simulink model "LQR_Controller"  (R2020b)
settings: Solver=VariableStepAuto  StartTime=0.0  StopTime=10.0  RelTol=1e-3
settings Model: Creator=24365  LastModifiedBy=24365

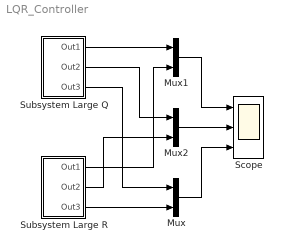
== system LQR_Controller ==
  Mux : Mux  Inputs=2
  Mux1 : Mux  Inputs=2
  Mux2 : Mux  Inputs=2
  Scope : Scope  NumInputPorts=3
  Subsystem Large Q : Subsystem
  Subsystem Large R : Subsystem
  wires:
  Subsystem Large Q/1(Out1) -> Mux1/1
  Subsystem Large Q/2(Out2) -> Mux2/1
  Subsystem Large Q/3(Out3) -> Mux/1
  Subsystem Large R/1(Out1) -> Mux1/2
  Subsystem Large R/2(Out2) -> Mux2/2
  Subsystem Large R/3(Out3) -> Mux/2
  Mux1/1 -> Scope/1
  Mux2/1 -> Scope/2
  Mux/1 -> Scope/3

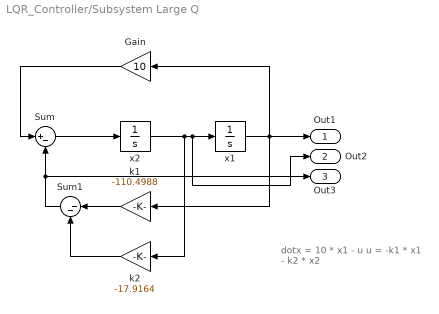
== system LQR_Controller/Subsystem Large Q ==
  note: dotx = 10 * x1 - u
      | u = -k1 * x1 - k2 * x2
  Gain : Gain  Gain=10
  Sum : Sum  Inputs=|+-
  Sum1 : Sum  Inputs=|--
  k1 : Gain  Gain=-110.4988
  k2 : Gain  Gain=-17.9164
  x1 : Integrator  InitialCondition=5
  x2 : Integrator
  Out1 : Outport
  Out2 : Outport  Port=2
  Out3 : Outport  Port=3
  wires:
  x2/1 -> k2/1, Out2/1, x1/1
  Sum1/1 -> Out3/1, Sum/2
  k2/1 -> Sum1/2
  k1/1 -> Sum1/1
  Gain/1 -> Sum/1
  x1/1 -> Out1/1, k1/1, Gain/1
  Sum/1 -> x2/1

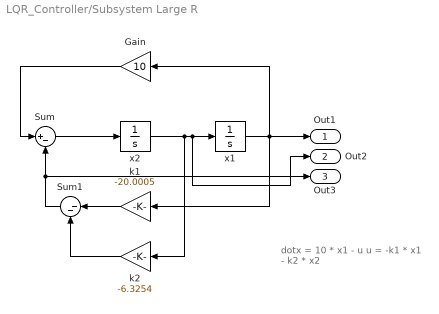
== system LQR_Controller/Subsystem Large R ==
  note: dotx = 10 * x1 - u
      | u = -k1 * x1 - k2 * x2
  Gain : Gain  Gain=10
  Sum : Sum  Inputs=|+-
  Sum1 : Sum  Inputs=|--
  k1 : Gain  Gain=-20.0005
  k2 : Gain  Gain=-6.3254
  x1 : Integrator  InitialCondition=5
  x2 : Integrator
  Out1 : Outport
  Out2 : Outport  Port=2
  Out3 : Outport  Port=3
  wires:
  x2/1 -> k2/1, Out2/1, x1/1
  Sum1/1 -> Out3/1, Sum/2
  k2/1 -> Sum1/2
  k1/1 -> Sum1/1
  Gain/1 -> Sum/1
  x1/1 -> Out1/1, k1/1, Gain/1
  Sum/1 -> x2/1
